simulink model "Model_Uebung_4"  (R2021a)
settings: Solver=VariableStepAuto  StartTime=0.0  StopTime=stop_time  RelTol=1e-3
values from neighbouring files (symbols this model uses):
  A = 1 + a1*q1 + a2*q2    [ableitung.m]    (also in init_4.m = [1 -1.6 0.64]; ubung4.m = [1 -1.6 0.64])
  B = b    [ableitung.m]    (also in init_4.m = 0.15; ubung4.m = 0.15)
  C = 1 - c*q1    [ableitung.m]    (also in init_4.m = 0.5; ubung4.m = [1 -0.5])
  Delta = 1    [init_4.m]    (also in ubung4.m; uebung_04.m; uebung_04_pram.m)
  step_time = stop_time    (= 6000)    [init_4.m]
  Theta0 = [-1.3 0.8 0.3 -0.3]    [init_4.m]    (also in ubung4.m = [-1.3 0.8 0.3 -0.3]')
undefined symbols (not defined in the file or in its folder): P0
settings Model: Creator=Tomo  LastModifiedBy=Tomo

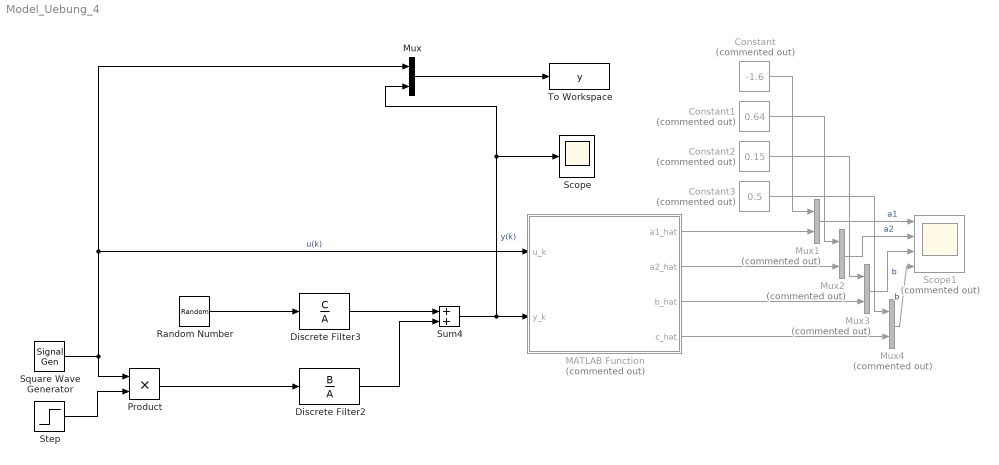
== system Model_Uebung_4 ==
  Constant : Constant  Commented=on  Value=-1.6
  Constant1 : Constant  Commented=on  Value=0.64
  Constant2 : Constant  Commented=on  Value=0.15
  Constant3 : Constant  Commented=on  Value=0.5
  Discrete Filter2 : DiscreteFilter  Numerator=B  Denominator=A  SampleTime=Delta
  Discrete Filter3 : DiscreteFilter  Numerator=C  Denominator=A  SampleTime=Delta
  MATLAB Function : MATLAB Function  Commented=on  TreatAsAtomicUnit=on  SystemSampleTime=Delta
  Mux : Mux  Inputs=2
  Mux{1..4} (4 alike) : Mux  Commented=on  Inputs=2
  Product : Product
  Random Number : RandomNumber  Variance=0.1^2  SampleTime=Delta
  Scope : Scope
  Scope1 : Scope  Commented=on  NumInputPorts=4
  Square Wave Generator : SignalGenerator  WaveForm=square  Frequency=0.01
  Step : Step  Time=step_time  Before=1  After=2  SampleTime=0
  Sum4 : Sum
  To Workspace : ToWorkspace  VariableName=y  SaveFormat=Timeseries  SampleTime=-1
  wires:
  Square Wave Generator/1 -> MATLAB Function/1(u_k), Mux/1, Product/1  "u(k)"
  Step/1 -> Product/2
  Product/1 -> Discrete Filter2/1
  Random Number/1 -> Discrete Filter3/1
  Discrete Filter3/1 -> Sum4/1
  Discrete Filter2/1 -> Sum4/2
  Sum4/1 -> Mux/2, Scope/1, MATLAB Function/2(y_k)  "y(k)"
  Mux2/1 -> Scope1/2  "a2"
  Constant1/1 -> Mux2/1
  Constant/1 -> Mux1/1
  Constant2/1 -> Mux3/1
  MATLAB Function/2(a2_hat) -> Mux2/2
  MATLAB Function/1(a1_hat) -> Mux1/2
  Mux1/1 -> Scope1/1  "a1"
  Mux3/1 -> Scope1/3  "b"
  MATLAB Function/3(b_hat) -> Mux3/2
  MATLAB Function/4(c_hat) -> Mux4/2
  Constant3/1 -> Mux4/1
  Mux4/1 -> Scope1/4  "b"
  Mux/1 -> To Workspace/1

== matlab function Model_Uebung_4/MATLAB Function ==
  data: u_k input; y_k input; P0 parameter; Theta0 parameter; a1_hat output; a2_hat output; b_hat output; c_hat output
function [a1_hat, a2_hat, b_hat, c_hat] = fcn(u_k, y_k, P0, Theta0)
    d = 2;
    lambda = 0.995;
    alpha_k = 1;
    
    persistent theta_hat y_hat J
    if isempty(y_hat)
        step = 0;
        P_k = P0;
        theta_hat = Theta0';
        u = zeros(1, d);
        y = zeros(1, d);
    end
    step = step + 1;
    if step>d
        phi = [u(end-d+1) -y(end) -y(end-1)]';
        L = P_k * phi / (lambda/alpha_k + phi' * P_k * phi);
        theta_hat = theta_hat + L * (y_k - phi' * theta_hat);
        P_k = 1 / lambda * (P_k - L * phi' * P_k);
        
        u = [u(2:end) u_k];
        y = [y(2:end) y_k];
    else
        u(step) = u_k;
        y(step) = y_k;
    end
    
    J = 0.5 * (y_k - y_hat)^2 + J;
    dJ = - (y_k - y_hat)*dy;
    
    a1_hat = theta_hat(1);
    a2_hat = theta_hat(2);
    b_hat = theta_hat(3);
    c_hat = theta_hat(4);
end
